simulink model "verify_Saturation_Property_mdl"  (R2018b)
settings: Solver=VariableStepDiscrete  StartTime=0.0  StopTime=6  MaxStep=1  RelTol=1e-3  EnableMultiTasking=on
libraries: carnot x1
settings Model: Creator=drhf  LastModifiedBy=drhf
settings DataIOCC: LimitDataPoints=on  SaveFormat=Array
settings OptimizationCC: ExpressionDepthLimit=2147483647  LifeSpan=inf
settings DebuggingCC: UnderspecifiedInitializationDetection=Classic  MergeDetectMultiDrivingBlocksExec=none  SolverPrmCheckMsg=warning  StateNameClashWarn=warning  SFUnexpectedBacktrackingDiag=warning  SFNoUnconditionalDefaultTransitionDiag=warning  SFExecutionAtInitializationDiag=none
settings HardwareCC: ProdBitPerPointer=32  ProdBitPerSizeT=32  ProdBitPerPtrDiffT=32  ProdLargestAtomicFloat=None  ProdIntDivRoundTo=Undefined  ProdEndianess=Unspecified  ProdWordSize=32  ProdHWDeviceType=32-bit Generic
settings ModelReferenceCC: PropagateSignalLabelsOutOfModel=off
settings SFSimCC: SimUseLocalCustomCode=off
settings RTWCC: RTWUseLocalCustomCode=off
settings CodeAppCC: StateflowObjectComments=on
settings GRTTargetCC: TargetLangStandard=C89/C90 (ANSI)  GeneratePreprocessorConditionals=Disable all  CombineOutputUpdateFcns=off  GRTInterface=on
settings ConfigComp: CovMetricSettings=dw  CovHtmlReporting=on  CovSaveCumulativeToWorkspaceVar=on  CovSaveSingleToWorkspaceVar=on  CovExternalEMLEnable=off

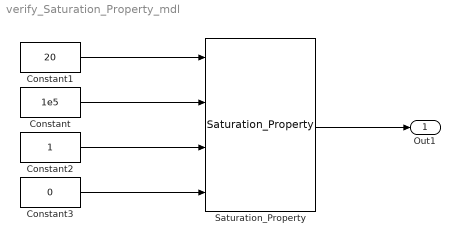
== system verify_Saturation_Property_mdl ==
  Constant : Constant  Value=1e5
  Constant1 : Constant  Value=20
  Constant2 : Constant
  Constant3 : Constant  Value=0
  Saturation_Property : carnot/Basic/Material_Properties/Saturation_Property  VariantControl=CarlibClassic  INPUTARGUMENTS=state variables (classic)  PROPERTY=density  FLUIDPHASE=liquid  DEBUGLEVEL=WARNINGLEVEL  MAXTOTALMESSAGES=inf  MAXCONSECUTIVEMESSAGES=inf  WRITETOFILE=0  FILENAME='errors.txt'
  Out1 : Outport
  wires:
  Saturation_Property/1 -> Out1/1
  Constant/1 -> Saturation_Property/2
  Constant1/1 -> Saturation_Property/1
  Constant2/1 -> Saturation_Property/3
  Constant3/1 -> Saturation_Property/4
